simulink model "sensors_static_test"  (R2018b)
settings: Solver=FixedStepAuto  StartTime=0.0  StopTime=10.0  RelTol=1e-3
libraries: gyroscope_lib x1, magnetometer_lib x1, solar_panels_lib x1, sun_sensor_lib x1
settings Model: Creator=Taylor  LastModifiedBy=Taylor

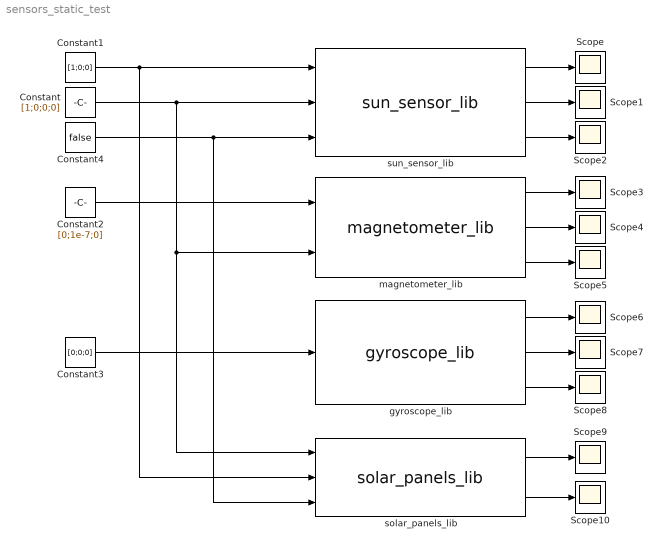
== system sensors_static_test ==
  Constant : Constant  Value=[1;0;0;0]
  Constant1 : Constant  Value=[1;0;0]
  Constant2 : Constant  Value=[0;1e-7;0]
  Constant3 : Constant  Value=[0;0;0]
  Constant4 : Constant  Value=false  OutDataTypeStr=boolean
  Scope{,1..10} (11 alike) : Scope
  gyroscope_lib : gyroscope_lib/gyroscope_lib  id_s=1
  magnetometer_lib : magnetometer_lib/magnetometer_lib  id_s=1
  solar_panels_lib : solar_panels_lib/solar_panels_lib  SystemSampleTime=-1
  "sun_sensor_lib " : sun_sensor_lib/sun_sensor_lib   SystemSampleTime=-1
  wires:
  Constant/1 -> solar_panels_lib/1, magnetometer_lib/2, "sun_sensor_lib "/2
  Constant1/1 -> solar_panels_lib/2, "sun_sensor_lib "/1
  Constant2/1 -> magnetometer_lib/1
  Constant3/1 -> gyroscope_lib/1
  "sun_sensor_lib "/1 -> Scope/1
  "sun_sensor_lib "/2 -> Scope1/1
  "sun_sensor_lib "/3 -> Scope2/1
  magnetometer_lib/1 -> Scope3/1
  magnetometer_lib/2 -> Scope4/1
  magnetometer_lib/3 -> Scope5/1
  gyroscope_lib/1 -> Scope6/1
  gyroscope_lib/2 -> Scope7/1
  gyroscope_lib/3 -> Scope8/1
  solar_panels_lib/1 -> Scope9/1
  solar_panels_lib/2 -> Scope10/1
  Constant4/1 -> solar_panels_lib/3, "sun_sensor_lib "/3
